simulink model "BF_sans_controleur_analyse"  (R2021b)
settings: Solver=VariableStepAuto  StartTime=0.0  StopTime=10.0  RelTol=1e-3
values from neighbouring files (symbols this model uses):
  A = [0 0 0  1 0 0   0 0 0   0 0 0 ... (first row only)    [systune_constant_gain_LPV.m]    (also in systune_gain_scheduling.m)
  B = [0 0 0 0 ... (first row only)    [systune_constant_gain_LPV.m]    (also in systune_gain_scheduling.m)
  B2 = [0 0 ... (first row only)    [systune_constant_gain_LPV.m]    (also in systune_gain_scheduling.m)
  C = eye(12)    [systune_constant_gain_LPV.m]    (also in systune_gain_scheduling.m)
  C_control = [1 0 0 0 0 0 0 0 0 0 0 0 ... (132 elements, 11x12)]    [matrix_systune.mat]    (also in systune_constant_gain_LPV.m = [C(1:7,:);C(9:12,:)]; systune_gain_scheduling.m = [C(1:7,:);C(9:12,:)])
  D = zeros(12,6)    [systune_constant_gain_LPV.m]    (also in systune_gain_scheduling.m)
  F = [1  0; 1  0; 0  1; 0  1]    [matrix_systune.mat]    (also in systune_constant_gain_LPV.m = [1 0; 1 0; 0 1; 0 1]; systune_gain_scheduling.m = [1 0; 1 0; 0 1; 0 1])
  H_val = [-0.0932839971064 -0.42306476603 1.20759628683 0.232835292684 0.261145596766 0.0874543759906 0.499376325725 -0.683953641731 4.19689639754 0.781501381691 0.946246535714 0.293513373789 ... (22 elements, 2x11)]    [matrix_systune.mat]    (also in systune_constant_gain_LPV.m = H_val.D; systune_gain_scheduling.m = H_val.D)
  K_val = [0.347835684479 0.322486277754 0.0964358277709 0.0893486830204 -0.165944108363 0.0623768203941 -0.0223487919109 0.0303550515766 -0.136766787558 -0.12376081504 0.00244423607368 0.0147163225433 ... (44 elements, 4x11)]    [matrix_systune.mat]    (also in systune_constant_gain_LPV.m = K_val.D; systune_gain_scheduling.m = K_val.D)
  x_12 = [[0; 0; 0]; [0; 0; 0]; [0; sin(angle/2); 0]; [0; 0; 0]]    [systune_constant_gain_LPV.m]    (also in systune_gain_scheduling.m)
settings Model: Creator=florian  LastModifiedBy=florian

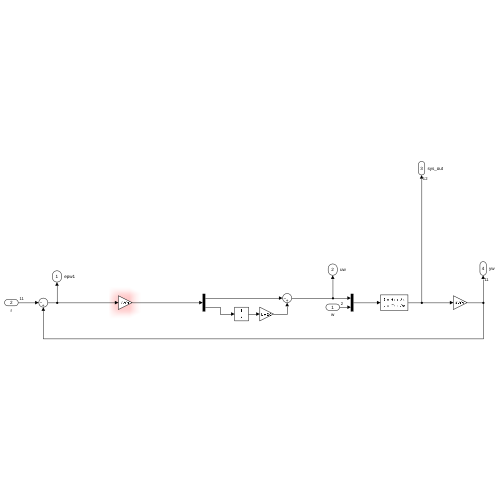
[thumbnail: Simulink's stored preview of the top-level diagram]
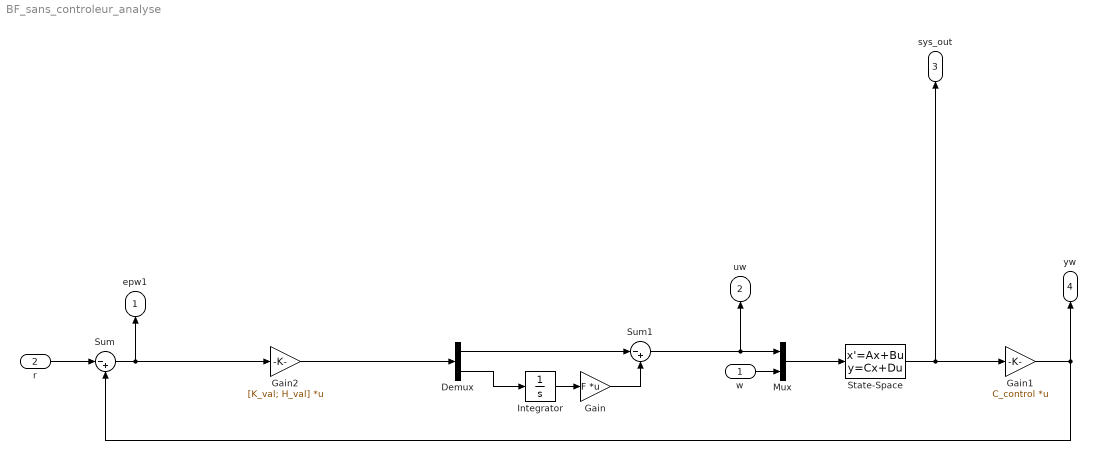
== system BF_sans_controleur_analyse ==
  w : Inport  PortDimensions=2
  r : Inport  Port=2  PortDimensions=11
  Demux : Demux  Outputs=2
  Gain : Gain  Gain=F  Multiplication=Matrix(K*u) (u vector)
  Gain1 : Gain  Gain=C_control  Multiplication=Matrix(K*u) (u vector)
  Gain2 : Gain  Gain=[K_val; H_val]  Multiplication=Matrix(K*u) (u vector)
  Integrator : Integrator
  Mux : Mux  Inputs=2
  State-Space : StateSpace  A=A  B=[B, B2]  C=C  D=D  InitialCondition=x_12
  Sum : Sum  Inputs=|-+
  Sum1 : Sum  Inputs=|-+
  epw1 : Outport  InitialOutput=0
  uw : Outport  Port=2  InitialOutput=0
  sys_out : Outport  Port=3  PortDimensions=12
  yw : Outport  Port=4  PortDimensions=11
  wires:
  Demux/2 -> Integrator/1
  Sum1/1 -> uw/1, Mux/1
  Sum/1 -> Gain2/1, epw1/1
  Gain2/1 -> Demux/1
  State-Space/1 -> Gain1/1, sys_out/1
  Gain/1 -> Sum1/2
  w/1 -> Mux/2
  Gain1/1 -> yw/1, Sum/2
  Demux/1 -> Sum1/1
  Mux/1 -> State-Space/1
  r/1 -> Sum/1
  Integrator/1 -> Gain/1
